simulink model "power_3levelVSC"  (Simulink 6.0)
settings: Solver=FixedStepDiscrete  SolverMode=SingleTasking  StartTime=0.0  StopTime=0.15  FixedStep=Ts_Power  RelTol=1e-3
InitFcn:
  | Ts_Power=5e-6;
  | Ts_Control=100e-6;
  | load power_3levelVSC_xinit
undefined symbols (not defined in the file or in its folder): D1, Delta, level
libraries: powerlib_extras x18, powerlib x16, simulink_extras x1
settings Model: Creator=Gilbert Sybille, IREQ  LastModifiedBy=batserve  ExtModeTrigMode=oneshot  ExtModeArmWhenConnect=off  ExtModeAutoUpdateStatusClock=off  ProdHWDeviceType=Specified
settings DataIOCC: LimitDataPoints=off  LoadInitialState=on  SaveFormat=StructureWithTime  SaveOutput=off  SaveTime=off  SignalLoggingName=sigsOut
settings OptimizationCC: BlockReduction=off  BooleanDataType=off
settings DebuggingCC: SolverPrmCheckMsg=none
settings HardwareCC: ProdBitPerShort=32  ProdBitPerInt=16  ProdHWDeviceType=Specified  TargetUnknown=on

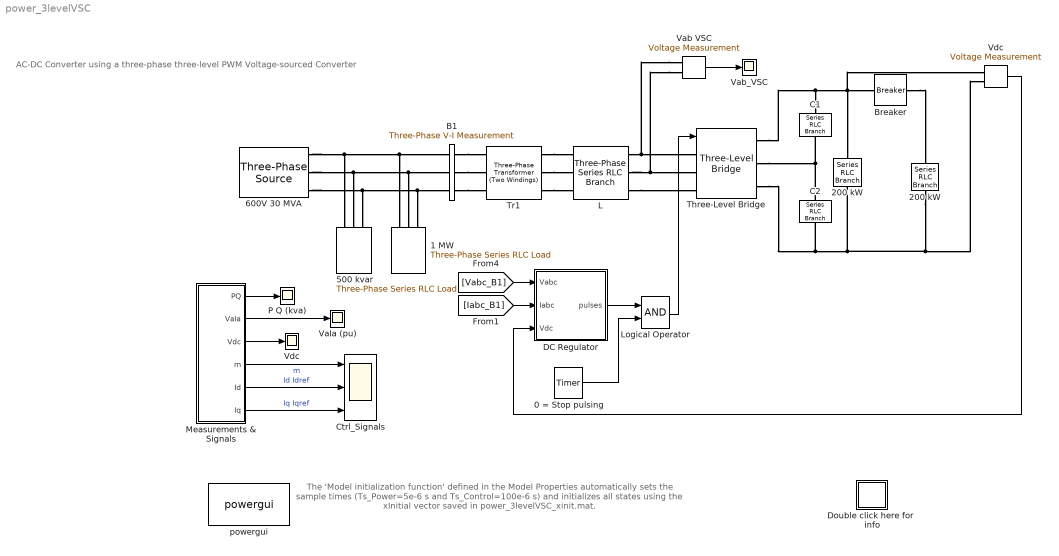
== system power_3levelVSC ==
  note: AC-DC Converter using a three-phase three-level
      | PWM Voltage-sourced Converter
  note: The 'Model  initialization function' defined in the
      | Model Properties automatically sets the
      | sample times (Ts_Power=5e-6 s and Ts_Control=100e-6 s)
      | and initializes all states using the xInitial vector saved
      | in power_3levelVSC_xinit.mat.
  0 = Stop pulsing : powerlib_extras/Control  Blocks/Timer  t=[0 0.1]  e=[1 0]
  1 MW : powerlib/Elements/Three-Phase Series RLC Load  Orientation=down  PhysicalDomain=powersysdomain  SubClassName=unknown  LeftPortType=p1  RightPortType=p1  LConnTagsString=A|B|C  Configuration=Y (grounded)  NominalVoltage=600  NominalFrequency=60  ActivePower=1e6  InductivePower=0  CapacitivePower=0  Measurements=None
  200 kW : powerlib/Elements/Series RLC Branch  Orientation=down  PhysicalDomain=powersysdomain  SubClassName=unknown  LeftPortType=p1  RightPortType=p1  LConnTagsString=__new0  RConnTagsString=__new0  Resistance=500^2/200e3  Inductance=0  Capacitance=inf  Measurements=None
  "200 kW " : powerlib/Elements/Series RLC Branch  Orientation=down  PhysicalDomain=powersysdomain  SubClassName=unknown  LeftPortType=p1  RightPortType=p1  LConnTagsString=__new0  RConnTagsString=__new0  Resistance=500^2/200e3  Inductance=0  Capacitance=inf  Measurements=None
  500 kvar : powerlib/Elements/Three-Phase Series RLC Load  Orientation=down  PhysicalDomain=powersysdomain  SubClassName=unknown  LeftPortType=p1  RightPortType=p1  LConnTagsString=A|B|C  Configuration=Y (grounded)  NominalVoltage=600  NominalFrequency=60  ActivePower=0.5e6/100  InductivePower=0  CapacitivePower=0.5e6  Measurements=None
  600V 30 MVA : powerlib/Electrical Sources/Three-Phase Source  Voltage=600  PhaseAngle=0  Frequency=60  InternalConnection=Yg  SpecifyImpedance=on  Resistance=0.724  Inductance=19.2e-3  ShortCircuitLevel=30e6  BaseVoltage=600  XRratio=10
  B1 : powerlib/Measurements/Three-Phase V-I Measurement  VoltageMeasurement=phase-to-ground  SetLabelV=on  LabelV=Vabc_B1  Vpu=off  Vbase=500e3  CurrentMeasurement=yes  SetLabelI=on  LabelI=Iabc_B1  Ipu=off  Pbase=100e6  OutputType=Magnitude  PhasorSimulation=off  PSBequivalent=0
  Breaker : powerlib/Elements/Breaker  BreakerResistance=0.001  InitialState=0  SnubberResistance=1e6  SnubberCapacitance=inf  SwitchingTimes=[0.05]  External=off  Measurements=None
      settings: AttributesFormatString=\n
  C1 : powerlib/Elements/Series RLC Branch  Orientation=down  PhysicalDomain=powersysdomain  SubClassName=unknown  LeftPortType=p1  RightPortType=p1  LConnTagsString=__new0  RConnTagsString=__new0  Resistance=0  Inductance=0  Capacitance=75000e-06  Measurements=None
  C2 : powerlib/Elements/Series RLC Branch  Orientation=down  PhysicalDomain=powersysdomain  SubClassName=unknown  LeftPortType=p1  RightPortType=p1  LConnTagsString=__new0  RConnTagsString=__new0  Resistance=0  Inductance=0  Capacitance=75000e-06  Measurements=None
  Ctrl_Signals : Scope  NumInputPorts=3
      settings: TimeRange=0.15  YMin=0.2~-0.5~-0.3  YMax=1~1.5~0.1  SaveName=V_Load  DataFormat=Array  SampleInput=on  SampleTime=Ts_Control
  DC Regulator : Subsystem  mask(DC Voltage Regulator){Vdc_Ref=500}
      mask prompts: Vdc_Ref "DC voltage setpoint (V):"
  Double click here for  info : Subsystem
      mask Type: Information
      mask Display: disp('?')
  L : powerlib/Elements/Three-Phase Series RLC Branch  PhysicalDomain=powersysdomain  SubClassName=unknown  LeftPortType=p1  RightPortType=p1  LConnTagsString=A|B|C  RConnTagsString=A|B|C  Resistance=0.1e-3  Inductance=20e-6  Capacitance=inf  Measurements=None
  Logical Operator : Logic  AllPortsSameDT=off  OutDataTypeMode=Specify via dialog  LogicDataType=float('double')
  Measurements & Signals : Subsystem
  P Q (kva) : Scope
      settings: YMin=-25  YMax=425  SaveName=PQ  DataFormat=Array  SampleInput=on  SampleTime=Ts_Control
  Three-Level Bridge : powerlib/Power Electronics/Three-Level Bridge  Arms=3  SnubberResistance=50  SbubberCapacitance=1e-6  Device=IGBT / Diodes  Ron=0.2e-3  ForwardVoltages="[  2 1 ]"  Measurements=All voltages and currents
  Tr1 : powerlib/Elements/Three-Phase Transformer (Two Windings)  NominalPower=[ 500e3 , 60 ]  Winding1Connection=Yg  Winding1=[ 600 , 0.04/30/2 , 0.04 ]  Winding2Connection=Delta (D1)  Winding2=[ 240 , 0.04/30/2 , 0.0 ]  SetSaturation=off  Rm=500  Lm=500  Saturation=[ 0,0 ; 0.0024,1.2 ; 1.0,1.52 ]  Hysteresis=off  DataFile='hysteresis'  SetInitialFlux=off  InitialFluxes=[ 0.8 , -0.8 , 0.7 ]  Measurements=None  TransfoNumber=0
  VaIa (pu) : Scope
      settings: TimeRange=0.15  YMin=-1.5  YMax=1.5  SaveName=VaIa  SampleInput=on  SampleTime=Ts_Power*2
  Vab VSC : powerlib/Measurements/Voltage Measurement  Tag=PoWeRsYsTeMmEaSuReMeNt  PhasorSimulation=off  OutputType=Magnitude  PSBequivalent=0
  Vab_VSC : Scope
      settings: TimeRange=0.05  YMin=-550  YMax=550  SaveName=Vab_VSC  SampleInput=on  SampleTime=Ts_Power
  Vdc : Scope
      settings: YMin=200  YMax=600  SaveName=Vdc  DataFormat=Array  SampleInput=on  SampleTime=Ts_Control
  "Vdc " : powerlib/Measurements/Voltage Measurement  Tag=PoWeRsYsTeMmEaSuReMeNt  PhasorSimulation=off  OutputType=Magnitude  PSBequivalent=0
  powergui : powerlib/powergui  Priority=2  Frange=logspace(0,3,50)  Ylog=off  Xlog=off  save=off  variable=ZData  structure=VaIa  ZoomFFT=on  StartTime=0.2  cycles=2  DisplayStyle=1  fundamental=60  FreqAxis=off  MaxFrequency=1000  frequencyindice=1  frequencyindicesteady=1  RmsSteady=2  display=off  Ts=Ts_Power  methode=off  frequency=60  echomessages=off
  wires:
  0 = Stop pulsing/1 -> Logical Operator/2
  DC Regulator/1(pulses) -> Logical Operator/1
  Measurements & Signals/1(PQ) -> P Q (kva)/1
  Measurements & Signals/2(VaIa) -> VaIa (pu)/1
  Measurements & Signals/3(Vdc) -> Vdc/1
  Measurements & Signals/4(m) -> Ctrl_Signals/1  "m"
  Measurements & Signals/5(Id) -> Ctrl_Signals/2  "Id Idref"
  Measurements & Signals/6(Iq) -> Ctrl_Signals/3  "Iq Iqref"
  [Vabc_B1] -> DC Regulator/1(Vabc)
  [Iabc_B1] -> DC Regulator/2(Iabc)
  Vab VSC/1 -> Vab_VSC/1
  "Vdc "/1 -> DC Regulator/3(Vdc)
  Logical Operator/1 -> Three-Level Bridge/1
  connections:
  600V 30 MVA/RConn1 -- B1/LConn1 -- 1 MW/LConn1 -- 500 kvar/LConn1
  600V 30 MVA/RConn2 -- B1/LConn2 -- 1 MW/LConn2 -- 500 kvar/LConn2
  600V 30 MVA/RConn3 -- B1/LConn3 -- 1 MW/LConn3 -- 500 kvar/LConn3
  Tr1/RConn1 -- L/LConn1
  Tr1/RConn2 -- L/LConn2
  Tr1/RConn3 -- L/LConn3
  Vab VSC/LConn1 -- L/RConn1 -- Three-Level Bridge/LConn1
  Vab VSC/LConn2 -- L/RConn2 -- Three-Level Bridge/LConn2
  L/RConn3 -- Three-Level Bridge/LConn3
  Three-Level Bridge/RConn1 -- "Vdc "/LConn1 -- Breaker/LConn1 -- 200 kW/LConn1 -- C1/LConn1
  Breaker/RConn1 -- "200 kW "/LConn1
  B1/RConn1 -- Tr1/LConn1
  B1/RConn2 -- Tr1/LConn2
  B1/RConn3 -- Tr1/LConn3
  C2/LConn1 -- C1/RConn1 -- Three-Level Bridge/RConn2
  "200 kW "/RConn1 -- Three-Level Bridge/RConn3 -- C2/RConn1 -- 200 kW/RConn1 -- "Vdc "/LConn2

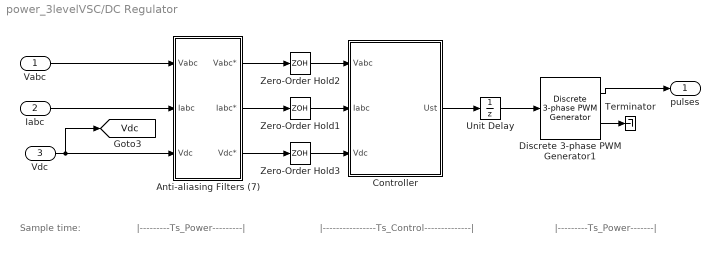
== system power_3levelVSC/DC Regulator ==
  note: |----------------Ts_Control--------------|
  note: |---------Ts_Power---------|
  note: Sample time:
  note: |---------Ts_Power-------|
  Vabc : Inport  Port=1  PortDimensions=3  LatchInput=off
  Iabc : Inport  Port=2  PortDimensions=3  LatchInput=off
  Vdc : Inport  Port=3  PortDimensions=1  LatchInput=off
  Anti-aliasing Filters (7) : Subsystem  mask(Anti-aliasing (2nd order lowpass)){Fc=750, Ts=Ts_Power}
      mask prompts: Fc "Cut-off frequency (Hz):"; Ts "Sample time:"
  Controller : Subsystem  mask(DC Regulator){Vdc_Ref=Vdc_Ref, Par_VdcReg=[0.015 1.6], Par_IReg=[0.3 20], Par_Nom=[600 500e3], Ts=Ts_Control}
      mask prompts: Vdc_Ref "DC Voltage setpoint (Volts)"; Par_VdcReg "Vdc Regulator Gains: [ Kp  Ki ]"; Par_IReg "Current Regulators Gain: [ Kp Ki Kd ]"; Par_Nom "Nominal Voltage and power: [ Vnom (volts rms L-L)  Pnom (VA) ]"; Ts "Time Step (s)"
      mask init:
      | Vnom=Par_Nom(1);
      | Pnom=Par_Nom(2);
      | Kp_I=Par_IReg(1);
      | Ki_I=Par_IReg(2);
      | Kp_Vdc=Par_VdcReg(1);
      | Ki_Vdc=Par_VdcReg(2);
  Discrete 3-phase PWM Generator1 : powerlib_extras/Discrete  Control Blocks/Discrete 3-phase PWM Generator  ModulatorType=3-level  ModulatorMode=Un-synchronized  nF=18  Fc=27*60  ModulatingSignals=off  m=0.2  Freq=60  Phase=0  Ts=Ts_Power
  Terminator : Terminator
  Unit Delay : UnitDelay  SampleTime=Ts_Control
  Zero-Order Hold1 : ZeroOrderHold  SampleTime=Ts_Control
  Zero-Order Hold2 : ZeroOrderHold  SampleTime=Ts_Control
  Zero-Order Hold3 : ZeroOrderHold  SampleTime=Ts_Control
  pulses : Outport
  tag scope: Vdc=global
  wires:
  Discrete 3-phase PWM Generator1/2 -> Terminator/1
  Discrete 3-phase PWM Generator1/1 -> pulses/1
  Unit Delay/1 -> Discrete 3-phase PWM Generator1/1
  Controller/1(Ust) -> Unit Delay/1
  Anti-aliasing Filters (7)/1(" Vabc*") -> Zero-Order Hold2/1
  Anti-aliasing Filters (7)/2(Iabc*) -> Zero-Order Hold1/1
  Anti-aliasing Filters (7)/3(" Vdc*") -> Zero-Order Hold3/1
  Zero-Order Hold3/1 -> Controller/3(Vdc)
  Zero-Order Hold1/1 -> Controller/2(Iabc)
  Zero-Order Hold2/1 -> Controller/1(Vabc)
  Vdc/1 -> [Vdc], Anti-aliasing Filters (7)/3("Vdc ")
  Iabc/1 -> Anti-aliasing Filters (7)/2("Iabc ")
  Vabc/1 -> Anti-aliasing Filters (7)/1(Vabc)

== system power_3levelVSC/Double click here for  info ==
  note: The DC regulator  uses two PI regulators to control the DC voltage while maintaining a unity input
      | power factor for the AC supply.
  note: 4) Controller:
  note: 2) AC Supply: three-phase, 600 V, 30 MVA, 60 Hz system
  note: 1) Converter rating: 500 Volts DC, 500 kW
  note: - DC Link: 2 capacitors of 75000 uF
  note: - Three-level, three-phase IGBT bridge (modeled using the "Three-Level Bridge" block)
      | controlled by a PWM modulator (carrier frequency of 1620 Hz)
  note: 3) Voltage-sourced Converter (VSC):
  note: Model Description:
  note: - In the simulation (lasting 150 ms), we can observe the following signals:
  note: Simulation Description:
  note: - Initial conditions set at the start of the simulation (by automatically loading the file: psb3levelVSC_xinit.mat prior to the simulation).
      | This file has been generated by running an initial simulation to steady-state for an integer number of cycles of 60 Hz.
      | The final states (both SimPowerSystems and Simulink controllers states)  were saved in a vector, called xInitial. This vector,
      | as well as the sample times (Ts_Power and Ts_Control) were saved in "power_3levelVSC_xinit.mat" file.
  note: Ts_Control= 100 us (used for the simulation of the DC regulator)
  note: - Two sample times: Ts_Power= 5 us (used by PSB for the simulation of the power system + converters)
  note: - Discrete (no continous states)
  note: AC-DC Converter
      | using a three-phase three-level PWM Voltage-sourced Converter
  note: Simulation Parameters:
  note: This AC-DC Converter demo illustrates the operation of the Three-Level Bridge block .
  note: P. Giroux ; G. Sybille Hydro-Quebec (IREQ)
  note: 1) the DC voltage (Vdc Scope)
      | 2) the primary voltage and current (phase A) of the AC supply (VaIa Scope),
      | 3) the device currents of leg A of the IGBT bridge (double-click inside the "Measurements & Signals" block to look inside the "Ia_Devices" Scope).
      | 4) the phase-to-phase AC voltage generated by the VSC (Vab_VSC Scope)
  note: - At 100 ms,  a "Stop Pulsing" signal is activated (pulses normally sent to the converter are blocked). We can see that the
      | DC voltage drops to 315 V. A drastic change in the primary current waveform can also be observed.
      | When the pulses are blocked, the Three-Level Bridge block operation becomes similar to a three-phase diode bridge.
  note: - At 50 ms, a 200-kW load is switched-in. We can see that the dynamic response of the DC regulator to this sudden load
      | variation (200 kW to 400 kW) is satisfactory. The DC voltage is back to 500 V within 1.5 cycle and the unity power factor
      | on the AC side is maintained.

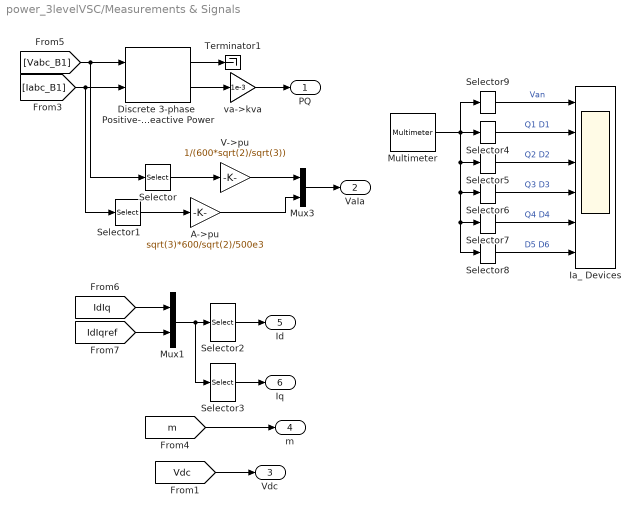
== system power_3levelVSC/Measurements & Signals ==
  A->pu : Gain  Gain=sqrt(3)*600/sqrt(2)/500e3  SaturateOnIntegerOverflow=on
  Discrete 3-phase  Positive-Sequence  Active & Reactive Power : powerlib_extras/Discrete Measurements/Discrete 3-phase  Positive-Sequence  Active & Reactive Power  Freq=60  Par_Vinit=[370 0]  Par_Iinit=[5 0]  Ts=Ts_Power
  Ia_ Devices : Scope  NumInputPorts=6
      settings: TimeRange=0.033  YMin=-400~-0~-0~0~0~0  YMax=300~7500~7500~4000~4000~7500  SaveName=I_Q3_disc1  DataFormat=Array  SampleInput=on  SampleTime=Ts_Power*2
  Multimeter : powerlib/Measurements/Multimeter  Tag=PoWeRsYsTeMmEaSuReMeNt  PhasorSimulation=off  OutputType=Magnitude  sel=[1 6 7 8 9 10 11 12 13 14 15]  L=35  Gain=[1 1 1 1 1 1 1 1 1 1 1]  yselected={'Uan: Three-Level Bridge','IQ1a: Three-Level Bridge','IQ2a: Three-Level Bridge','IQ3a: Three-Level Bridge','IQ4a: Three-Level Bridge','ID1a: Three-Level Bridge','ID2a: Three-Level Bridge','ID3a: Three-Level Bridge','ID4a: Three-Level Bridge','ID5a: Three-Level Bridge','ID6a: Three-Level Bridge'};  PSBOutputType=1  PSBequivalent=0  AxesSetting=[0,0.1,-100,100]  Display=0  SavedBlockNames=-11
      settings: AttributesFormatString=\n
  Mux1 : Mux  Inputs=2
  Mux3 : Mux  Inputs=2
  Selector : Selector  InputPortWidth=3
  Selector1 : Selector  InputPortWidth=3
  Selector2 : Selector  Elements=[1 3]  InputPortWidth=4
  Selector3 : Selector  Elements=[1 3]+1  InputPortWidth=4
  Selector4 : Selector  Elements=[1 5]+1  InputPortWidth=11
  Selector5 : Selector  Elements=[1 5]+2  InputPortWidth=11
  Selector6 : Selector  Elements=[1 5]+3  InputPortWidth=11
  Selector7 : Selector  Elements=[1 5]+4  InputPortWidth=11
  Selector8 : Selector  Elements=[10 11]  InputPortWidth=11
  Selector9 : Selector  InputPortWidth=11
  Terminator1 : Terminator
  V->pu : Gain  Gain=1/(600*sqrt(2)/sqrt(3))  SaturateOnIntegerOverflow=on
  va->kva : Gain  Gain=1e-3  SaturateOnIntegerOverflow=on
  PQ : Outport
  VaIa : Outport  Port=2
  Vdc : Outport  Port=3
  m : Outport  Port=4
  Id : Outport  Port=5
  Iq : Outport  Port=6
  wires:
  va->kva/1 -> PQ/1
  Selector8/1 -> Ia_ Devices/6  "D5 D6"
  Selector7/1 -> Ia_ Devices/5  "Q4 D4"
  Selector6/1 -> Ia_ Devices/4  "Q3 D3"
  Selector5/1 -> Ia_ Devices/3  "Q2 D2"
  Selector4/1 -> Ia_ Devices/2  "Q1 D1"
  Selector9/1 -> Ia_ Devices/1  "Van"
  A->pu/1 -> Mux3/2
  V->pu/1 -> Mux3/1
  Selector3/1 -> Iq/1
  Selector2/1 -> Id/1
  [m] -> m/1
  Mux1/1 -> Selector3/1, Selector2/1
  [Vdc] -> Vdc/1
  Mux3/1 -> VaIa/1
  Discrete 3-phase  Positive-Sequence  Active & Reactive Power/2 -> va->kva/1
  Discrete 3-phase  Positive-Sequence  Active & Reactive Power/1 -> Terminator1/1
  [Iabc_B1] -> Selector1/1, Discrete 3-phase  Positive-Sequence  Active & Reactive Power/2
  [Vabc_B1] -> Selector/1, Discrete 3-phase  Positive-Sequence  Active & Reactive Power/1
  Selector1/1 -> A->pu/1
  Selector/1 -> V->pu/1
  [IdIqref] -> Mux1/2
  [IdIq] -> Mux1/1
  Multimeter/1 -> Selector9/1, Selector8/1, Selector7/1, Selector6/1, Selector5/1, Selector4/1

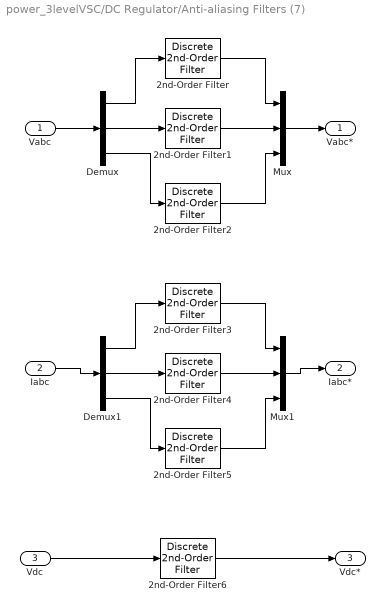
== system power_3levelVSC/DC Regulator/Anti-aliasing Filters (7) ==
  Vabc : Inport  Port=1  PortDimensions=3  LatchInput=off
  "Iabc " : Inport  Port=2  PortDimensions=3  LatchInput=off
  "Vdc " : Inport  Port=3  PortDimensions=1  LatchInput=off
  2nd-Order Filter : powerlib_extras/Discrete  Control Blocks/Discrete  2nd-Order Filter  FilterType=Lowpass  Fo=Fc  Zeta=0.707  Ts=Ts  Initialize=off  Vac_Init=[0.8 -25 60]  Vdc_Init=-0.4  PlotResponse=off  param1=[1 2000 0.2]
  2nd-Order Filter{1..2,4..6} (5 alike) : powerlib_extras/Discrete  Control Blocks/Discrete  2nd-Order Filter  FilterType=Lowpass  Fo=Fc  Zeta=0.707  Ts=Ts  Initialize=off  Vac_Init=[0.8 -25 60]  Vdc_Init=-0.4  PlotResponse=off  param1=[1 5000 0.1]
  2nd-Order Filter3 : powerlib_extras/Discrete  Control Blocks/Discrete  2nd-Order Filter  FilterType=Lowpass  Fo=Fc  Zeta=0.707  Ts=Ts  Initialize=off  Vac_Init=[0.8 -25 60]  Vdc_Init=-0.4  PlotResponse=off  param1=[1 2000 0.2]
  Demux : Demux  Outputs=3
  Demux1 : Demux  Outputs=3
  Mux : Mux  Inputs=3
  Mux1 : Mux  Inputs=3
  " Vabc*" : Outport
  Iabc* : Outport  Port=2
  " Vdc*" : Outport  Port=3
  wires:
  Mux1/1 -> Iabc*/1
  Demux1/2 -> 2nd-Order Filter4/1
  Demux1/3 -> 2nd-Order Filter5/1
  2nd-Order Filter5/1 -> Mux1/3
  2nd-Order Filter4/1 -> Mux1/2
  2nd-Order Filter3/1 -> Mux1/1
  Demux1/1 -> 2nd-Order Filter3/1
  "Iabc "/1 -> Demux1/1
  Demux/2 -> 2nd-Order Filter1/1
  Demux/3 -> 2nd-Order Filter2/1
  2nd-Order Filter2/1 -> Mux/3
  2nd-Order Filter1/1 -> Mux/2
  2nd-Order Filter6/1 -> " Vdc*"/1
  "Vdc "/1 -> 2nd-Order Filter6/1
  Mux/1 -> " Vabc*"/1
  2nd-Order Filter/1 -> Mux/1
  Vabc/1 -> Demux/1
  Demux/1 -> 2nd-Order Filter/1

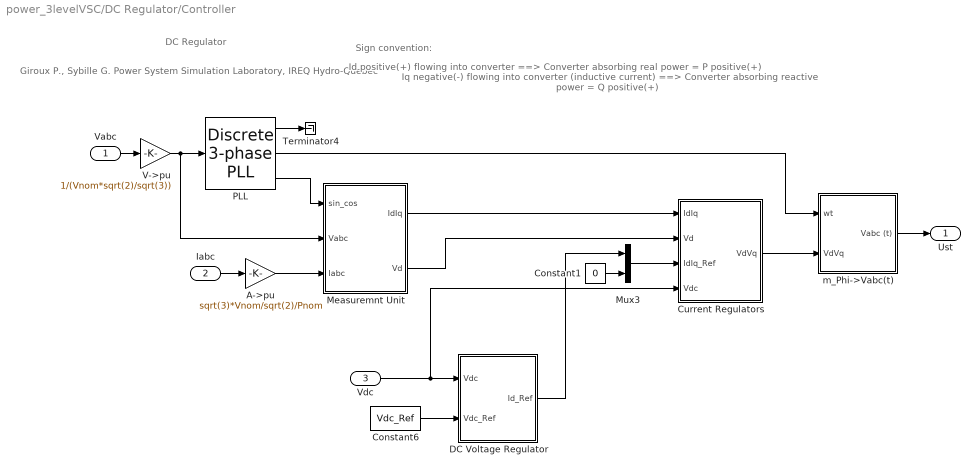
== system power_3levelVSC/DC Regulator/Controller ==
  note: DC Regulator
  note: Giroux P., Sybille G.
      | Power System Simulation Laboratory, IREQ
      | Hydro-Quebec
  note: Iq negative(-) flowing into converter (inductive current) ==> Converter absorbing reactive power = Q positive(+)
  note: Sign convention:
  note: Id positive(+) flowing into converter ==> Converter absorbing real power = P positive(+)
  Vabc : Inport  Port=1  PortDimensions=3  LatchInput=off
  Iabc : Inport  Port=2  PortDimensions=3  LatchInput=off
  Vdc : Inport  Port=3  PortDimensions=1  LatchInput=off
  A->pu : Gain  Gain=sqrt(3)*Vnom/sqrt(2)/Pnom  SaturateOnIntegerOverflow=on
  Constant1 : Constant  Value=0
  Constant6 : Constant  Value=Vdc_Ref
  Current Regulators : Subsystem  mask(Current Regulators){Kp=Kp_I, Ki=Ki_I, Kd=0, TcD=0.2e-3, Par_Limits=[12 -12], Init=0, Ts=Ts}
      mask prompts: Kp "Proportional gain (Kp):"; Ki "Integral gain (Ki):"; Kd "Derivative gain (Kd):"; TcD "Time constant for derivative (s):"; Par_Limits "Output limits: [ Upper   Lower ]"; Init "Output initial value:"; Ts "Sample time:"
      mask help:
      | Sign convention:
      | Id positive(+) flowing into converter ==> Converter absorbing real power = P positive(+)
      | Iq negative(-) flowing into converter (inductive current) ==> Converter absorbing reactive power = Q positive(+)
  DC Voltage Regulator : Subsystem  mask(DC Voltage regulator){Kp=Kp_Vdc, Ki=Ki_Vdc, Ts=Ts}
      mask prompts: Kp "Proportional gain (Kp):"; Ki "Integral gain(Ki)"; Ts "Sample time:"
  Measuremnt Unit : Subsystem
  Mux3 : Mux  Inputs=2
  PLL : powerlib_extras/Discrete  Control Blocks/Discrete 3-phase PLL  Fmin=45  Par_Init=[-45 60]  ParK=[60 1400]  Ts=Ts
  Terminator4 : Terminator
  V->pu : Gain  Gain=1/(Vnom*sqrt(2)/sqrt(3))  SaturateOnIntegerOverflow=on
  m_Phi->Vabc(t) : Subsystem
  Ust : Outport
  wires:
  m_Phi->Vabc(t)/1(Vabc (t)) -> Ust/1
  PLL/2 -> m_Phi->Vabc(t)/1(wt)
  Current Regulators/1(VdVq) -> m_Phi->Vabc(t)/2(VdVq)
  DC Voltage Regulator/1(Id_Ref) -> Mux3/1
  Constant1/1 -> Mux3/2
  Mux3/1 -> Current Regulators/3(IdIq_Ref)
  Measuremnt Unit/2(Vd) -> Current Regulators/2(Vd)
  Measuremnt Unit/1(IdIq) -> Current Regulators/1(IdIq)
  Iabc/1 -> A->pu/1
  PLL/3 -> Measuremnt Unit/1(sin_cos)
  PLL/1 -> Terminator4/1
  Vdc/1 -> Current Regulators/4(Vdc), DC Voltage Regulator/1(Vdc)
  Constant6/1 -> DC Voltage Regulator/2(Vdc_Ref)
  Vabc/1 -> V->pu/1
  V->pu/1 -> PLL/1, Measuremnt Unit/2(Vabc)
  A->pu/1 -> Measuremnt Unit/3(Iabc)

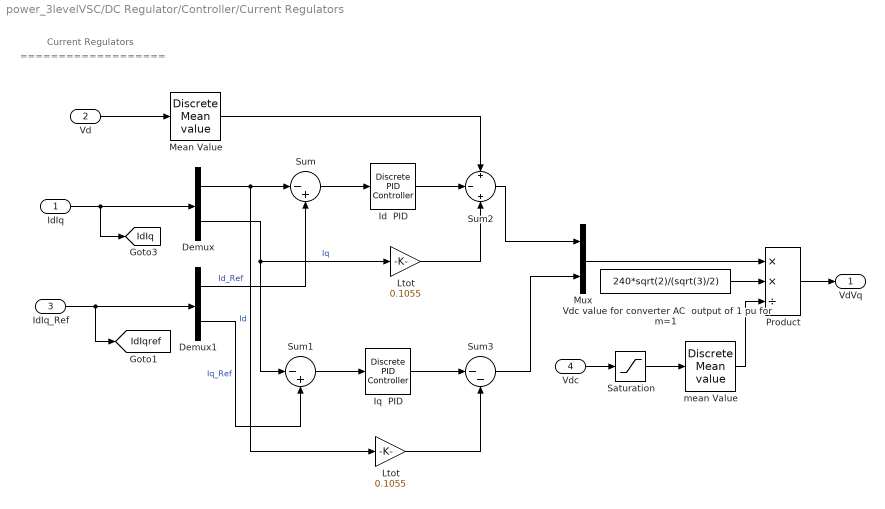
== system power_3levelVSC/DC Regulator/Controller/Current Regulators ==
  note: ===================
  note: Current Regulators
  IdIq : Inport  Port=1  PortDimensions=2  LatchInput=off
  Vd : Inport  Port=2  LatchInput=off
  IdIq_Ref : Inport  Port=3  PortDimensions=2  LatchInput=off
  Vdc : Inport  Port=4  LatchInput=off
  " Ltot" : Gain  Gain=0.1055  SaturateOnIntegerOverflow=on
  Demux : Demux  Outputs=2
  Demux1 : Demux  Outputs=2
  Id  PID : powerlib_extras/Discrete  Control Blocks/Discrete PID Controller  Kp=Kp  Ki=Ki  Kd=Kd  TcD=TcD  Par_Limits=Par_Limits  Init=Init  Ts=Ts
  Iq  PID : powerlib_extras/Discrete  Control Blocks/Discrete PID Controller  Kp=Kp  Ki=Ki  Kd=Kd  TcD=TcD  Par_Limits=Par_Limits  Init=Init  Ts=Ts
  "Ltot " : Gain  Gain=0.1055  SaturateOnIntegerOverflow=on
  Mean Value : powerlib_extras/Discrete Measurements/Discrete  Mean value  Freq=60  Vinit=1.007  Ts=Ts
  Mux : Mux  Inputs=2
  Product : Product  Inputs=**/  SaturateOnIntegerOverflow=on  InputSameDT=on
  Saturation : Saturate  UpperLimit=10000  LowerLimit=10
  Sum : Sum  Inputs=|-+  SaturateOnIntegerOverflow=on  InputSameDT=on
  Sum1 : Sum  Inputs=|-+  SaturateOnIntegerOverflow=on  InputSameDT=on
  Sum2 : Sum  Inputs=+|-|+  SaturateOnIntegerOverflow=on  InputSameDT=on
  Sum3 : Sum  Inputs=|--  SaturateOnIntegerOverflow=on  InputSameDT=on
  Vdc value for converter AC  output of 1 pu for m=1 : Constant  Value=240*sqrt(2)/(sqrt(3)/2)
  "mean Value " : powerlib_extras/Discrete Measurements/Discrete  Mean value  Freq=60  Vinit=500  Ts=Ts
  VdVq : Outport
  tag scope: IdIq=global, IdIqref=global
  wires:
  Sum3/1 -> Mux/2
  Vdc/1 -> Saturation/1
  "mean Value "/1 -> Product/3
  Vdc value for converter AC  output of 1 pu for m=1/1 -> Product/2
  Saturation/1 -> "mean Value "/1
  Mean Value/1 -> Sum2/1
  Product/1 -> VdVq/1
  IdIq_Ref/1 -> [IdIqref], Demux1/1
  Mux/1 -> Product/1
  Sum/1 -> Id  PID/1
  Demux1/2 -> Sum1/2  "Iq_Ref"
  Sum1/1 -> Iq  PID/1
  Demux/2 -> Sum1/1, "Ltot "/1  "Iq"
  Demux1/1 -> Sum/2  "Id_Ref"
  Demux/1 -> " Ltot"/1, Sum/1  "Id"
  IdIq/1 -> [IdIq], Demux/1
  Id  PID/1 -> Sum2/2
  Sum2/1 -> Mux/1
  Iq  PID/1 -> Sum3/1
  "Ltot "/1 -> Sum2/3
  " Ltot"/1 -> Sum3/2
  Vd/1 -> Mean Value/1

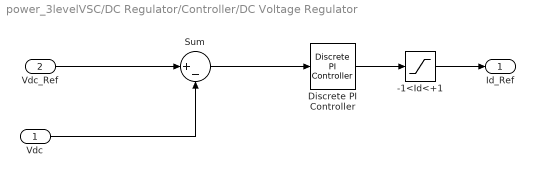
== system power_3levelVSC/DC Regulator/Controller/DC Voltage Regulator ==
  Vdc : Inport  Port=1  LatchInput=off
  Vdc_Ref : Inport  Port=2  LatchInput=off
  -1<Id<+1 : Saturate  UpperLimit=1.2  LowerLimit=-1.2
  Discrete PI Controller : powerlib_extras/Discrete  Control Blocks/Discrete PI Controller  Kp=Kp  Ki=Ki  Par_Limits=[1.2 -1.2]  Init=0  Ts=Ts
  Sum : Sum  Inputs=|+-  SaturateOnIntegerOverflow=on  InputSameDT=on
  Id_Ref : Outport  InitialOutput=0
  wires:
  Sum/1 -> Discrete PI Controller/1
  Vdc/1 -> Sum/2
  Discrete PI Controller/1 -> -1<Id<+1/1
  -1<Id<+1/1 -> Id_Ref/1
  Vdc_Ref/1 -> Sum/1

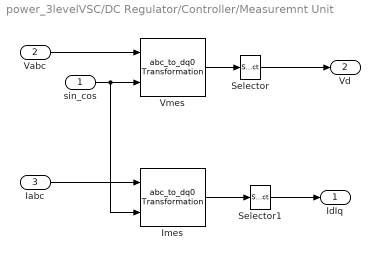
== system power_3levelVSC/DC Regulator/Controller/Measuremnt Unit ==
  sin_cos : Inport  Port=1  LatchInput=off
  Vabc : Inport  Port=2  LatchInput=off
  Iabc : Inport  Port=3  LatchInput=off
  Imes : powerlib_extras/Measurements/abc_to_dq0 Transformation
  Selector : Selector  InputPortWidth=3
  Selector1 : Selector  Elements=[1 2]  InputPortWidth=3
  Vmes : powerlib_extras/Measurements/abc_to_dq0 Transformation
  IdIq : Outport
  Vd : Outport  Port=2
  wires:
  Selector/1 -> Vd/1
  Imes/1 -> Selector1/1
  Iabc/1 -> Imes/1
  sin_cos/1 -> Imes/2, Vmes/2
  Vmes/1 -> Selector/1
  Vabc/1 -> Vmes/1
  Selector1/1 -> IdIq/1

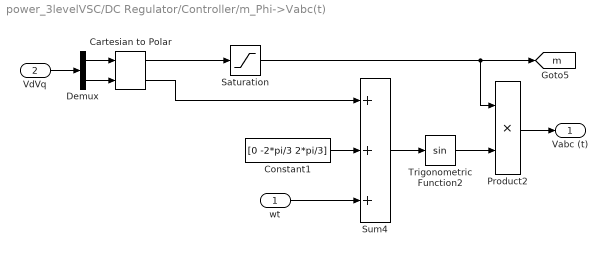
== system power_3levelVSC/DC Regulator/Controller/m_Phi->Vabc(t) ==
  wt : Inport  Port=1  LatchInput=off
  VdVq : Inport  Port=2  LatchInput=off
  Cartesian to Polar : simulink_extras/Transformations/Cartesian to Polar
  Constant1 : Constant  Value=[0 -2*pi/3 2*pi/3]
  Demux : Demux  Outputs=2
  Product2 : Product  SaturateOnIntegerOverflow=on  InputSameDT=on
  Saturation : Saturate  UpperLimit=1  LowerLimit=0
  Sum4 : Sum  Inputs=+++  SaturateOnIntegerOverflow=on  InputSameDT=on
  Trigonometric Function2 : Trigonometry
  Vabc (t) : Outport
  tag scope: m=global
  wires:
  Saturation/1 -> [m], Product2/1
  Cartesian to Polar/1 -> Saturation/1
  Trigonometric Function2/1 -> Product2/2
  Sum4/1 -> Trigonometric Function2/1
  Cartesian to Polar/2 -> Sum4/1
  Demux/2 -> Cartesian to Polar/2
  Demux/1 -> Cartesian to Polar/1
  VdVq/1 -> Demux/1
  wt/1 -> Sum4/3
  Product2/1 -> Vabc (t)/1
  Constant1/1 -> Sum4/2
